simulink model "case7"  (R2024b)
settings: Solver=FixedStepAuto  StartTime=0  StopTime=1  FixedStep=1e-7  RelTol=1e-3
values from neighbouring files (symbols this model uses):
  SG_D_1_D = 0.01056    [IEEE9_case_parameters.m]    (also in case1_parameters.m; case2_parameters.m; case3_parameters.m; case4_parameters.m)
  SG_D_1_EnableSaturation = 0    [IEEE9_case_parameters.m]    (also in case1_parameters.m; case2_parameters.m; case3_parameters.m; case4_parameters.m)
  SG_D_1_f0 = 60    [IEEE9_case_parameters.m]    (also in case1_parameters.m; case2_parameters.m; case3_parameters.m; case4_parameters.m)
  SG_D_1_H = 7.5    [IEEE9_case_parameters.m]    (also in case1_parameters.m; case2_parameters.m; case3_parameters.m; case4_parameters.m)
  SG_D_1_K_A = 20    [IEEE9_case_parameters.m]    (also in case1_parameters.m; case2_parameters.m; case3_parameters.m; case4_parameters.m)
  SG_D_1_K_E = 1.000000e+1    (= 10)    [IEEE9_case_parameters.m]    (also in case1_parameters.m; case2_parameters.m; case3_parameters.m; case4_parameters.m)
  SG_D_1_K_F = 2.363    [IEEE9_case_parameters.m]    (also in case1_parameters.m; case2_parameters.m; case3_parameters.m; case4_parameters.m)
  SG_D_1_K_s = 0.5    [IEEE9_case_parameters.m]    (also in case1_parameters.m = 5; case2_parameters.m = 5; case3_parameters.m = 5; case4_parameters.m = 5)
  SG_D_1_R_a = 0.001088    [IEEE9_case_parameters.m]    (also in case1_parameters.m; case2_parameters.m; case3_parameters.m; case4_parameters.m)
  SG_D_1_S_A = 1    [IEEE9_case_parameters.m]    (also in case1_parameters.m; case2_parameters.m; case3_parameters.m; case4_parameters.m)
  SG_D_1_S_B = 0.103    [IEEE9_case_parameters.m]    (also in case1_parameters.m; case2_parameters.m; case3_parameters.m; case4_parameters.m)
  SG_D_1_S_N = 10.659857    [IEEE9_case_parameters.m]    (also in case1_parameters.m; case2_parameters.m; case3_parameters.m; case4_parameters.m)
  SG_D_1_SpeedPara = 200    [IEEE9_case_parameters.m]    (also in case1_parameters.m; case2_parameters.m; case3_parameters.m; case4_parameters.m)
  SG_D_1_T_0 = 0.720173    [IEEE9_case_parameters.m]    (also in case1_parameters.m = 0.755522; case2_parameters.m = 0.808931; case3_parameters.m = 0.869402; case4_parameters.m = 0.729316)
  SG_D_1_T_1 = 0.3    [IEEE9_case_parameters.m]    (also in case1_parameters.m; case2_parameters.m; case3_parameters.m; case4_parameters.m)
  SG_D_1_T_2 = 0.05    [IEEE9_case_parameters.m]    (also in case1_parameters.m; case2_parameters.m; case3_parameters.m; case4_parameters.m)
  SG_D_1_T_3 = 0.02    [IEEE9_case_parameters.m]    (also in case1_parameters.m; case2_parameters.m; case3_parameters.m; case4_parameters.m)
  SG_D_1_T_4 = 0.005    [IEEE9_case_parameters.m]    (also in case1_parameters.m; case2_parameters.m; case3_parameters.m; case4_parameters.m)
  SG_D_1_T_A = 0.02    [IEEE9_case_parameters.m]    (also in case1_parameters.m; case2_parameters.m; case3_parameters.m; case4_parameters.m)
  SG_D_1_T_dd = 8.000000e+0    (= 8)    [IEEE9_case_parameters.m]    (also in case1_parameters.m; case2_parameters.m; case3_parameters.m; case4_parameters.m)
  SG_D_1_T_ddd = 0.04    [IEEE9_case_parameters.m]    (also in case1_parameters.m; case2_parameters.m; case3_parameters.m; case4_parameters.m)
  SG_D_1_T_E = 0.314    [IEEE9_case_parameters.m]    (also in case1_parameters.m; case2_parameters.m; case3_parameters.m; case4_parameters.m)
  SG_D_1_T_F = 0.35    [IEEE9_case_parameters.m]    (also in case1_parameters.m; case2_parameters.m; case3_parameters.m; case4_parameters.m)
  SG_D_1_T_qd = 0.8    [IEEE9_case_parameters.m]    (also in case1_parameters.m; case2_parameters.m; case3_parameters.m; case4_parameters.m)
  SG_D_1_T_qdd = 0.02    [IEEE9_case_parameters.m]    (also in case1_parameters.m; case2_parameters.m; case3_parameters.m; case4_parameters.m)
  SG_D_1_T_speed = 0.1    [IEEE9_case_parameters.m]    (also in case1_parameters.m = 200; case2_parameters.m = 200; case3_parameters.m = 200; case4_parameters.m = 200)
  SG_D_1_T_w = 0.5    [IEEE9_case_parameters.m]    (also in case1_parameters.m; case2_parameters.m; case3_parameters.m; case4_parameters.m)
  SG_D_1_V_ref = 1.990276    [IEEE9_case_parameters.m]    (also in case1_parameters.m = 2.042296; case2_parameters.m = 2.051388; case3_parameters.m = 2.089584; case4_parameters.m = 2.01845)
  SG_D_1_w_ref = 376.991118    [IEEE9_case_parameters.m]    (also in case1_parameters.m; case2_parameters.m; case3_parameters.m; case4_parameters.m)
  SG_D_1_wb = 6.000000e+1    (= 60)    [IEEE9_case_parameters.m]    (also in case1_parameters.m; case2_parameters.m; case3_parameters.m; case4_parameters.m)
  SG_D_1_x_d = 1.9    [IEEE9_case_parameters.m]    (also in case1_parameters.m; case2_parameters.m; case3_parameters.m; case4_parameters.m)
  SG_D_1_x_dd = 0.302    [IEEE9_case_parameters.m]    (also in case1_parameters.m; case2_parameters.m; case3_parameters.m; case4_parameters.m)
  SG_D_1_x_ddd = 0.204    [IEEE9_case_parameters.m]    (also in case1_parameters.m; case2_parameters.m; case3_parameters.m; case4_parameters.m)
  SG_D_1_x_l = 0.05    [IEEE9_case_parameters.m]    (also in case1_parameters.m; case2_parameters.m; case3_parameters.m; case4_parameters.m)
  SG_D_1_x_q = 1.3    [IEEE9_case_parameters.m]    (also in case1_parameters.m; case2_parameters.m; case3_parameters.m; case4_parameters.m)
  SG_D_1_x_qd = 0.5    [IEEE9_case_parameters.m]    (also in case1_parameters.m; case2_parameters.m; case3_parameters.m; case4_parameters.m)
  SG_D_1_x_qdd = 0.3    [IEEE9_case_parameters.m]    (also in case1_parameters.m; case2_parameters.m; case3_parameters.m; case4_parameters.m)
  SG_D_2_D = 0.02    [IEEE9_case_parameters.m]    (also in case1_parameters.m; case2_parameters.m; case3_parameters.m; case4_parameters.m)
  SG_D_2_EnableSaturation = 0    [IEEE9_case_parameters.m]    (also in case1_parameters.m; case2_parameters.m; case3_parameters.m; case4_parameters.m)
  SG_D_2_f0 = 60    [IEEE9_case_parameters.m]    (also in case1_parameters.m; case2_parameters.m; case3_parameters.m; case4_parameters.m)
  SG_D_2_H = 8.000000e+0    (= 8)    [IEEE9_case_parameters.m]    (also in case1_parameters.m; case2_parameters.m; case3_parameters.m; case4_parameters.m)
  SG_D_2_K_A = 20    [IEEE9_case_parameters.m]    (also in case1_parameters.m; case2_parameters.m; case3_parameters.m; case4_parameters.m)
  SG_D_2_K_E = 1.000000e+1    (= 10)    [IEEE9_case_parameters.m]    (also in case1_parameters.m; case2_parameters.m; case3_parameters.m; case4_parameters.m)
  SG_D_2_K_F = 2.363    [IEEE9_case_parameters.m]    (also in case1_parameters.m; case2_parameters.m; case3_parameters.m; case4_parameters.m)
  SG_D_2_K_s = 0.5    [IEEE9_case_parameters.m]    (also in case1_parameters.m = 4; case2_parameters.m = 4; case3_parameters.m = 4; case4_parameters.m = 4)
  SG_D_2_R_a = 0.001088    [IEEE9_case_parameters.m]    (also in case1_parameters.m; case2_parameters.m; case3_parameters.m; case4_parameters.m)
  SG_D_2_S_A = 1    [IEEE9_case_parameters.m]    (also in case1_parameters.m; case2_parameters.m; case3_parameters.m; case4_parameters.m)
  SG_D_2_S_B = 0.103    [IEEE9_case_parameters.m]    (also in case1_parameters.m; case2_parameters.m; case3_parameters.m; case4_parameters.m)
  SG_D_2_S_N = 10.659857    [IEEE9_case_parameters.m]    (also in case1_parameters.m; case2_parameters.m; case3_parameters.m; case4_parameters.m)
  SG_D_2_SpeedPara = 200    [IEEE9_case_parameters.m]    (also in case1_parameters.m; case2_parameters.m; case3_parameters.m; case4_parameters.m)
  SG_D_2_T_0 = 1.632913    [IEEE9_case_parameters.m]    (also in case1_parameters.m = 1.632925; case2_parameters.m = 1.632915; case3_parameters.m = 1.632914; case4_parameters.m = 1.632927)
  SG_D_2_T_1 = 0.2    [IEEE9_case_parameters.m]    (also in case1_parameters.m; case2_parameters.m; case3_parameters.m; case4_parameters.m)
  SG_D_2_T_2 = 0.05    [IEEE9_case_parameters.m]    (also in case1_parameters.m; case2_parameters.m; case3_parameters.m; case4_parameters.m)
  SG_D_2_T_3 = 0.02    [IEEE9_case_parameters.m]    (also in case1_parameters.m; case2_parameters.m; case3_parameters.m; case4_parameters.m)
  SG_D_2_T_4 = 0.005    [IEEE9_case_parameters.m]    (also in case1_parameters.m; case2_parameters.m; case3_parameters.m; case4_parameters.m)
  SG_D_2_T_A = 0.02    [IEEE9_case_parameters.m]    (also in case1_parameters.m; case2_parameters.m; case3_parameters.m; case4_parameters.m)
  SG_D_2_T_dd = 7.9    [IEEE9_case_parameters.m]    (also in case1_parameters.m; case2_parameters.m; case3_parameters.m; case4_parameters.m)
  SG_D_2_T_ddd = 0.04    [IEEE9_case_parameters.m]    (also in case1_parameters.m; case2_parameters.m; case3_parameters.m; case4_parameters.m)
  SG_D_2_T_E = 0.314    [IEEE9_case_parameters.m]    (also in case1_parameters.m; case2_parameters.m; case3_parameters.m; case4_parameters.m)
  SG_D_2_T_F = 0.35    [IEEE9_case_parameters.m]    (also in case1_parameters.m; case2_parameters.m; case3_parameters.m; case4_parameters.m)
  SG_D_2_T_qd = 0.8    [IEEE9_case_parameters.m]    (also in case1_parameters.m; case2_parameters.m; case3_parameters.m; case4_parameters.m)
  SG_D_2_T_qdd = 0.015    [IEEE9_case_parameters.m]    (also in case1_parameters.m; case2_parameters.m; case3_parameters.m; case4_parameters.m)
  SG_D_2_T_speed = 0.1    [IEEE9_case_parameters.m]    (also in case1_parameters.m = 150; case2_parameters.m = 150; case3_parameters.m = 150; case4_parameters.m = 150)
  SG_D_2_T_w = 0.35    [IEEE9_case_parameters.m]    (also in case1_parameters.m; case2_parameters.m; case3_parameters.m; case4_parameters.m)
  SG_D_2_V_ref = 2.58547    [IEEE9_case_parameters.m]    (also in case1_parameters.m = 2.597896; case2_parameters.m = 2.587136; case3_parameters.m = 2.586042; case4_parameters.m = 2.599679)
  SG_D_2_w_ref = 376.991118    [IEEE9_case_parameters.m]    (also in case1_parameters.m; case2_parameters.m; case3_parameters.m; case4_parameters.m)
  SG_D_2_wb = 6.000000e+1    (= 60)    [IEEE9_case_parameters.m]    (also in case1_parameters.m; case2_parameters.m; case3_parameters.m; case4_parameters.m)
  SG_D_2_x_d = 1.8    [IEEE9_case_parameters.m]    (also in case1_parameters.m; case2_parameters.m; case3_parameters.m; case4_parameters.m)
  SG_D_2_x_dd = 0.302    [IEEE9_case_parameters.m]    (also in case1_parameters.m; case2_parameters.m; case3_parameters.m; case4_parameters.m)
  SG_D_2_x_ddd = 0.204    [IEEE9_case_parameters.m]    (also in case1_parameters.m; case2_parameters.m; case3_parameters.m; case4_parameters.m)
  SG_D_2_x_l = 0.05    [IEEE9_case_parameters.m]    (also in case1_parameters.m; case2_parameters.m; case3_parameters.m; case4_parameters.m)
  SG_D_2_x_q = 1.25    [IEEE9_case_parameters.m]    (also in case1_parameters.m; case2_parameters.m; case3_parameters.m; case4_parameters.m)
  SG_D_2_x_qd = 0.5    [IEEE9_case_parameters.m]    (also in case1_parameters.m; case2_parameters.m; case3_parameters.m; case4_parameters.m)
  SG_D_2_x_qdd = 0.3    [IEEE9_case_parameters.m]    (also in case1_parameters.m; case2_parameters.m; case3_parameters.m; case4_parameters.m)
  SG_D_3_D = 0.02    [IEEE9_case_parameters.m]    (also in case1_parameters.m; case2_parameters.m; case3_parameters.m; case4_parameters.m)
  SG_D_3_EnableSaturation = 0    [IEEE9_case_parameters.m]    (also in case1_parameters.m; case2_parameters.m; case3_parameters.m; case4_parameters.m)
  SG_D_3_f0 = 60    [IEEE9_case_parameters.m]    (also in case1_parameters.m; case2_parameters.m; case3_parameters.m; case4_parameters.m)
  SG_D_3_H = 7.7    [IEEE9_case_parameters.m]    (also in case1_parameters.m; case2_parameters.m; case3_parameters.m; case4_parameters.m)
  SG_D_3_K_A = 20    [IEEE9_case_parameters.m]    (also in case1_parameters.m; case2_parameters.m; case3_parameters.m; case4_parameters.m)
  SG_D_3_K_E = 1.000000e+1    (= 10)    [IEEE9_case_parameters.m]    (also in case1_parameters.m; case2_parameters.m; case3_parameters.m; case4_parameters.m)
  SG_D_3_K_F = 2.363    [IEEE9_case_parameters.m]    (also in case1_parameters.m; case2_parameters.m; case3_parameters.m; case4_parameters.m)
  SG_D_3_K_s = 0.2    [IEEE9_case_parameters.m]    (also in case1_parameters.m = 2; case2_parameters.m = 2; case3_parameters.m = 2; case4_parameters.m = 2)
  SG_D_3_R_a = 0.001088    [IEEE9_case_parameters.m]    (also in case1_parameters.m; case2_parameters.m; case3_parameters.m; case4_parameters.m)
  SG_D_3_S_A = 1    [IEEE9_case_parameters.m]    (also in case1_parameters.m; case2_parameters.m; case3_parameters.m; case4_parameters.m)
  SG_D_3_S_B = 0.103    [IEEE9_case_parameters.m]    (also in case1_parameters.m; case2_parameters.m; case3_parameters.m; case4_parameters.m)
  SG_D_3_S_N = 10.659857    [IEEE9_case_parameters.m]    (also in case1_parameters.m; case2_parameters.m; case3_parameters.m; case4_parameters.m)
  SG_D_3_SpeedPara = 200    [IEEE9_case_parameters.m]    (also in case1_parameters.m; case2_parameters.m; case3_parameters.m; case4_parameters.m)
  SG_D_3_T_0 = 0.850788    [IEEE9_case_parameters.m]    (also in case1_parameters.m = 0.850786; case2_parameters.m = 0.850787; case3_parameters.m; case4_parameters.m = 0.850786)
  SG_D_3_T_1 = 0.2    [IEEE9_case_parameters.m]    (also in case1_parameters.m; case2_parameters.m; case3_parameters.m; case4_parameters.m)
  SG_D_3_T_2 = 0.05    [IEEE9_case_parameters.m]    (also in case1_parameters.m; case2_parameters.m; case3_parameters.m; case4_parameters.m)
  SG_D_3_T_3 = 0.02    [IEEE9_case_parameters.m]    (also in case1_parameters.m; case2_parameters.m; case3_parameters.m; case4_parameters.m)
  SG_D_3_T_4 = 0.005    [IEEE9_case_parameters.m]    (also in case1_parameters.m; case2_parameters.m; case3_parameters.m; case4_parameters.m)
  SG_D_3_T_A = 0.02    [IEEE9_case_parameters.m]    (also in case1_parameters.m; case2_parameters.m; case3_parameters.m; case4_parameters.m)
  SG_D_3_T_dd = 8.1    [IEEE9_case_parameters.m]    (also in case1_parameters.m; case2_parameters.m; case3_parameters.m; case4_parameters.m)
  SG_D_3_T_ddd = 0.04    [IEEE9_case_parameters.m]    (also in case1_parameters.m; case2_parameters.m; case3_parameters.m; case4_parameters.m)
  SG_D_3_T_E = 0.314    [IEEE9_case_parameters.m]    (also in case1_parameters.m; case2_parameters.m; case3_parameters.m; case4_parameters.m)
  SG_D_3_T_F = 0.35    [IEEE9_case_parameters.m]    (also in case1_parameters.m; case2_parameters.m; case3_parameters.m; case4_parameters.m)
  SG_D_3_T_qd = 0.8    [IEEE9_case_parameters.m]    (also in case1_parameters.m; case2_parameters.m; case3_parameters.m; case4_parameters.m)
  SG_D_3_T_qdd = 0.015    [IEEE9_case_parameters.m]    (also in case1_parameters.m; case2_parameters.m; case3_parameters.m; case4_parameters.m)
  SG_D_3_T_speed = 0.1    [IEEE9_case_parameters.m]    (also in case1_parameters.m = 180; case2_parameters.m = 180; case3_parameters.m = 180; case4_parameters.m = 180)
  SG_D_3_T_w = 0.4    [IEEE9_case_parameters.m]    (also in case1_parameters.m; case2_parameters.m; case3_parameters.m; case4_parameters.m)
  SG_D_3_V_ref = 1.892727    [IEEE9_case_parameters.m]    (also in case1_parameters.m = 1.906439; case2_parameters.m = 1.895535; case3_parameters.m = 1.892105; case4_parameters.m = 1.906598)
  SG_D_3_w_ref = 376.991118    [IEEE9_case_parameters.m]    (also in case1_parameters.m; case2_parameters.m; case3_parameters.m; case4_parameters.m)
  SG_D_3_wb = 6.000000e+1    (= 60)    [IEEE9_case_parameters.m]    (also in case1_parameters.m; case2_parameters.m; case3_parameters.m; case4_parameters.m)
  SG_D_3_x_d = 1.85    [IEEE9_case_parameters.m]    (also in case1_parameters.m; case2_parameters.m; case3_parameters.m; case4_parameters.m)
  SG_D_3_x_dd = 0.302    [IEEE9_case_parameters.m]    (also in case1_parameters.m; case2_parameters.m; case3_parameters.m; case4_parameters.m)
  SG_D_3_x_ddd = 0.204    [IEEE9_case_parameters.m]    (also in case1_parameters.m; case2_parameters.m; case3_parameters.m; case4_parameters.m)
  SG_D_3_x_l = 0.05    [IEEE9_case_parameters.m]    (also in case1_parameters.m; case2_parameters.m; case3_parameters.m; case4_parameters.m)
  SG_D_3_x_q = 1.2    [IEEE9_case_parameters.m]    (also in case1_parameters.m; case2_parameters.m; case3_parameters.m; case4_parameters.m)
  SG_D_3_x_qd = 0.5    [IEEE9_case_parameters.m]    (also in case1_parameters.m; case2_parameters.m; case3_parameters.m; case4_parameters.m)
  SG_D_3_x_qdd = 0.3    [IEEE9_case_parameters.m]    (also in case1_parameters.m; case2_parameters.m; case3_parameters.m; case4_parameters.m)
(part 1 of 12)
settings Model: Creator=Greg  LastModifiedBy=Greg

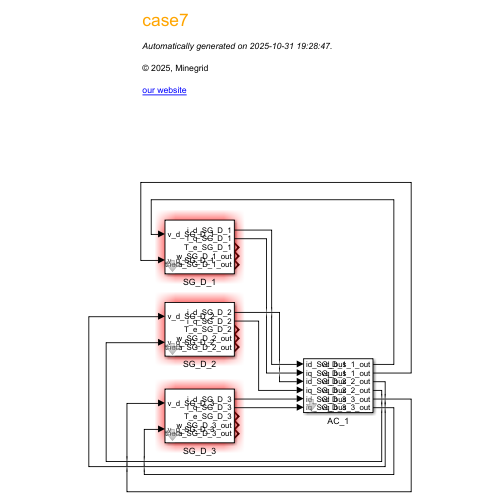
[thumbnail: Simulink's stored preview of the top-level diagram]
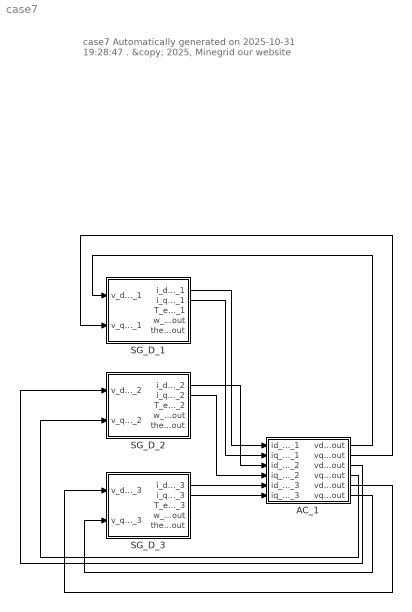
== system case7 ==
  note: case7
      | Automatically generated on 2025-10-31 19:28:47 .
      | &copy; 2025, Minegrid
      | our website
  AC_1 : Subsystem  mask(AC_1){}
      mask help: Parameters Interface of AC_1
  SG_D_1 : Subsystem  mask(SG_D_1){T_0=SG_D_1_T_0, w_ref=SG_D_1_w_ref, V_ref=SG_D_1_V_ref, x_d=SG_D_1_x_d, x_dd=SG_D_1_x_dd, x_ddd=SG_D_1_x_ddd, x_q=SG_D_1_x_q, x_qd=SG_D_1_x_qd, x_qdd=SG_D_1_x_qdd, x_l=SG_D_1_x_l, R_a=SG_D_1_R_a, T_dd=SG_D_1_T_dd, T_ddd=SG_D_1_T_ddd, T_qd=SG_D_1_T_qd, T_qdd=SG_D_1_T_qdd, H=SG_D_1_H, D=SG_D_1_D, SpeedPara=SG_D_1_SpeedPara, K_A=SG_D_1_K_A, EnableSaturation=SG_D_1_EnableSaturation, f0=SG_D_1_f0, T_speed=SG_D_1_T_speed, T_E=SG_D_1_T_E, T_A=SG_D_1_T_A, T_F=SG_D_1_T_F, K_E=SG_D_1_K_E, K_F=SG_D_1_K_F, K_s=SG_D_1_K_s, T_1=SG_D_1_T_1, T_2=SG_D_1_T_2, T_3=SG_D_1_T_3, T_4=SG_D_1_T_4, T_w=SG_D_1_T_w, wb=SG_D_1_wb, S_A=SG_D_1_S_A, S_B=SG_D_1_S_B, S_N=SG_D_1_S_N}
      mask help: Parameters Interface of SG_D_1
  SG_D_2 : Subsystem  mask(SG_D_2){T_0=SG_D_2_T_0, w_ref=SG_D_2_w_ref, V_ref=SG_D_2_V_ref, x_d=SG_D_2_x_d, x_dd=SG_D_2_x_dd, x_ddd=SG_D_2_x_ddd, x_q=SG_D_2_x_q, x_qd=SG_D_2_x_qd, x_qdd=SG_D_2_x_qdd, x_l=SG_D_2_x_l, R_a=SG_D_2_R_a, T_dd=SG_D_2_T_dd, T_ddd=SG_D_2_T_ddd, T_qd=SG_D_2_T_qd, T_qdd=SG_D_2_T_qdd, H=SG_D_2_H, D=SG_D_2_D, SpeedPara=SG_D_2_SpeedPara, K_A=SG_D_2_K_A, EnableSaturation=SG_D_2_EnableSaturation, f0=SG_D_2_f0, T_speed=SG_D_2_T_speed, T_E=SG_D_2_T_E, T_A=SG_D_2_T_A, T_F=SG_D_2_T_F, K_E=SG_D_2_K_E, K_F=SG_D_2_K_F, K_s=SG_D_2_K_s, T_1=SG_D_2_T_1, T_2=SG_D_2_T_2, T_3=SG_D_2_T_3, T_4=SG_D_2_T_4, T_w=SG_D_2_T_w, wb=SG_D_2_wb, S_A=SG_D_2_S_A, S_B=SG_D_2_S_B, S_N=SG_D_2_S_N}
      mask help: Parameters Interface of SG_D_2
  SG_D_3 : Subsystem  mask(SG_D_3){T_0=SG_D_3_T_0, w_ref=SG_D_3_w_ref, V_ref=SG_D_3_V_ref, x_d=SG_D_3_x_d, x_dd=SG_D_3_x_dd, x_ddd=SG_D_3_x_ddd, x_q=SG_D_3_x_q, x_qd=SG_D_3_x_qd, x_qdd=SG_D_3_x_qdd, x_l=SG_D_3_x_l, R_a=SG_D_3_R_a, T_dd=SG_D_3_T_dd, T_ddd=SG_D_3_T_ddd, T_qd=SG_D_3_T_qd, T_qdd=SG_D_3_T_qdd, H=SG_D_3_H, D=SG_D_3_D, SpeedPara=SG_D_3_SpeedPara, K_A=SG_D_3_K_A, EnableSaturation=SG_D_3_EnableSaturation, f0=SG_D_3_f0, T_speed=SG_D_3_T_speed, T_E=SG_D_3_T_E, T_A=SG_D_3_T_A, T_F=SG_D_3_T_F, K_E=SG_D_3_K_E, K_F=SG_D_3_K_F, K_s=SG_D_3_K_s, T_1=SG_D_3_T_1, T_2=SG_D_3_T_2, T_3=SG_D_3_T_3, T_4=SG_D_3_T_4, T_w=SG_D_3_T_w, wb=SG_D_3_wb, S_A=SG_D_3_S_A, S_B=SG_D_3_S_B, S_N=SG_D_3_S_N}
      mask help: Parameters Interface of SG_D_3
  wires:
  SG_D_2/2(i_q_SG_D_2) -> AC_1/4(iq_SG_D_2)
  SG_D_1/2(i_q_SG_D_1) -> AC_1/2(iq_SG_D_1)
  SG_D_1/1(i_d_SG_D_1) -> AC_1/1(id_SG_D_1)
  SG_D_2/1(i_d_SG_D_2) -> AC_1/3(id_SG_D_2)
  AC_1/1(vd_bus_1_out) -> SG_D_1/1(v_d_SG_D_1)
  SG_D_3/1(i_d_SG_D_3) -> AC_1/5(id_SG_D_3)
  AC_1/2(vq_bus_1_out) -> SG_D_1/2(v_q_SG_D_1)
  SG_D_3/2(i_q_SG_D_3) -> AC_1/6(iq_SG_D_3)
  AC_1/3(vd_bus_2_out) -> SG_D_2/1(v_d_SG_D_2)
  AC_1/4(vq_bus_2_out) -> SG_D_2/2(v_q_SG_D_2)
  AC_1/5(vd_bus_3_out) -> SG_D_3/1(v_d_SG_D_3)
  AC_1/6(vq_bus_3_out) -> SG_D_3/2(v_q_SG_D_3)

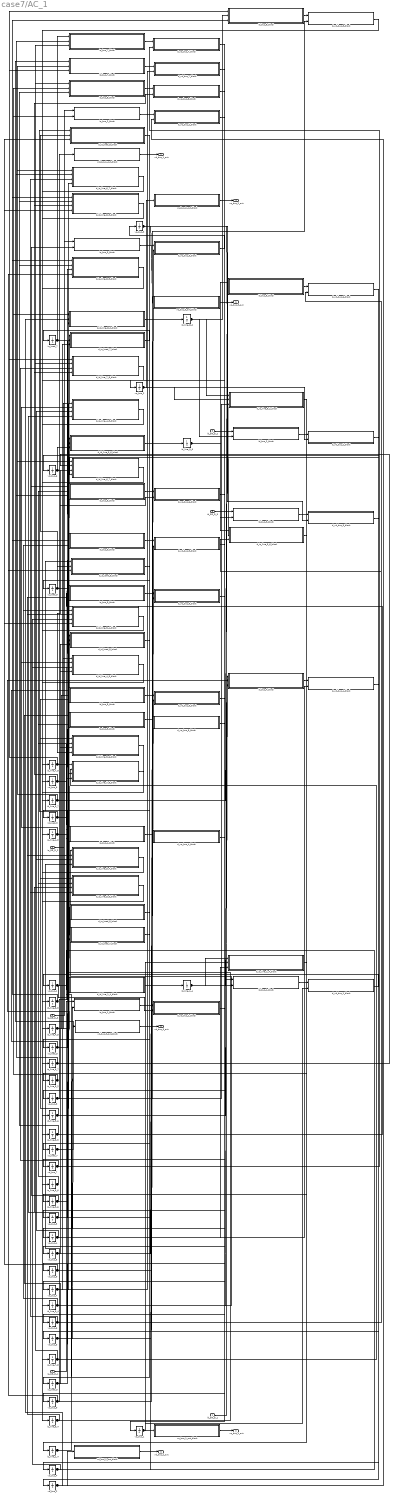
== system case7/AC_1 ==
  id_SG_D_1 : Inport
  iq_SG_D_1 : Inport  Port=2
  id_SG_D_2 : Inport  Port=3
  iq_SG_D_2 : Inport  Port=4
  id_SG_D_3 : Inport  Port=5
  iq_SG_D_3 : Inport  Port=6
  d_id_line_1_4_block : Subsystem
  d_id_line_3_6_block : Subsystem
  d_id_line_4_5_block : Subsystem
  d_id_line_5_6_block : Subsystem
  d_id_line_6_7_block : Subsystem
  d_id_line_7_8_block : Subsystem
  d_id_line_8_2_block : Subsystem
  d_id_line_8_9_block : Subsystem
  d_id_line_9_4_block : Subsystem
  d_id_load_5_block : Subsystem
  d_id_load_7_block : Subsystem
  d_id_load_9_block : Subsystem
  d_iq_line_1_4_block : Subsystem
  d_iq_line_3_6_block : Subsystem
  d_iq_line_4_5_block : Subsystem
  d_iq_line_5_6_block : Subsystem
  d_iq_line_6_7_block : Subsystem
  d_iq_line_7_8_block : Subsystem
  d_iq_line_8_2_block : Subsystem
  d_iq_line_8_9_block : Subsystem
  d_iq_line_9_4_block : Subsystem
  d_iq_load_5_block : Subsystem
  d_iq_load_7_block : Subsystem
  d_iq_load_9_block : Subsystem
  d_vd_bus_1_block : Subsystem
  d_vd_bus_2_block : Subsystem
  d_vd_bus_3_block : Subsystem
  d_vd_bus_4_block : Subsystem
  d_vd_bus_5_block : Subsystem
  d_vd_bus_6_block : Subsystem
  d_vd_bus_7_block : Subsystem
  d_vd_bus_8_block : Subsystem
  d_vd_bus_9_block : Subsystem
  d_vq_bus_1_block : Subsystem
  d_vq_bus_2_block : Subsystem
  d_vq_bus_3_block : Subsystem
  d_vq_bus_4_block : Subsystem
  d_vq_bus_5_block : Subsystem
  d_vq_bus_6_block : Subsystem
  d_vq_bus_7_block : Subsystem
  d_vq_bus_8_block : Subsystem
  d_vq_bus_9_block : Subsystem
  id_bus_1_block : Subsystem
  id_bus_2_block : Subsystem
  id_bus_3_block : Subsystem
  id_bus_4_block : Subsystem
  id_bus_5_block : Subsystem
  id_bus_6_block : Subsystem
  id_bus_7_block : Subsystem
  id_bus_8_block : Subsystem
  id_bus_9_block : Subsystem
  id_line_1_4 : Integrator  InitialCondition=0.7046
  id_line_3_6 : Integrator  InitialCondition=0.841
  id_line_4_5 : Integrator  InitialCondition=0.3014
  id_line_5_6 : Integrator  InitialCondition=-0.609
  id_line_6_7 : Integrator  InitialCondition=0.2421
  id_line_7_8 : Integrator  InitialCondition=-0.766
  id_line_8_2 : Integrator  InitialCondition=-1.6245
  id_line_8_9 : Integrator  InitialCondition=0.874
  id_line_9_4 : Integrator  InitialCondition=-0.3964
  id_load_5 : Integrator  InitialCondition=0.8929736913465931
  id_load_7 : Integrator  InitialCondition=1.0103745512612274
  id_load_9 : Integrator  InitialCondition=1.2530677383718292
  iq_bus_1_block : Subsystem
  iq_bus_2_block : Subsystem
  iq_bus_3_block : Subsystem
  iq_bus_4_block : Subsystem
  iq_bus_5_block : Subsystem
  iq_bus_6_block : Subsystem
  iq_bus_7_block : Subsystem
  iq_bus_8_block : Subsystem
  iq_bus_9_block : Subsystem
  iq_line_1_4 : Integrator  InitialCondition=-0.1877
  iq_line_3_6 : Integrator  InitialCondition=0.1412
  iq_line_4_5 : Integrator  InitialCondition=-0.0675
  iq_line_5_6 : Integrator  InitialCondition=0.0199
  iq_line_6_7 : Integrator  InitialCondition=-0.1237
  iq_line_7_8 : Integrator  InitialCondition=0.0069
  iq_line_8_2 : Integrator  InitialCondition=-0.1716
  iq_line_8_9 : Integrator  InitialCondition=-0.0481
  iq_line_9_4 : Integrator  InitialCondition=0.2855
  iq_load_5 : Integrator  InitialCondition=-0.3396268514243827
  iq_load_7 : Integrator  InitialCondition=-0.30769449147731925
  iq_load_9 : Integrator  InitialCondition=-0.5651600829422596
  vd_bus_1 : Integrator  InitialCondition=1.0
  vd_bus_1_out_block : Subsystem
  vd_bus_2 : Integrator  InitialCondition=0.9854656089996572
  vd_bus_2_out_block : Subsystem
  vd_bus_3 : Integrator  InitialCondition=0.9963648946924322
  vd_bus_3_out_block : Subsystem
  vd_bus_4 : Integrator  InitialCondition=0.9891468763636446
  vd_bus_5 : Integrator  InitialCondition=0.977867619882352
  vd_bus_6 : Integrator  InitialCondition=1.0046719033619074
  vd_bus_7 : Integrator  InitialCondition=0.9893152199851127
  vd_bus_8 : Integrator  InitialCondition=0.996231319283822
  vd_bus_9 : Integrator  InitialCondition=0.9608859398821573
  vq_bus_1 : Integrator  InitialCondition=0.0
  vq_bus_1_out_block : Subsystem
  vq_bus_2 : Integrator  InitialCondition=0.16987505255020435
  vq_bus_2_out_block : Subsystem
  vq_bus_3 : Integrator  InitialCondition=0.08518800751595623
  vq_bus_3_out_block : Subsystem
  vq_bus_4 : Integrator  InitialCondition=-0.040732947337366425
  vq_bus_5 : Integrator  InitialCondition=-0.06742985670686191
  vq_bus_6 : Integrator  InitialCondition=0.035721536791196516
  vq_bus_7 : Integrator  InitialCondition=0.012674842274998602
  vq_bus_8 : Integrator  InitialCondition=0.06797079213073709
  vq_bus_9 : Integrator  InitialCondition=-0.07173809262590466
  vd_bus_1_out : Outport
  vq_bus_1_out : Outport  Port=2
  vd_bus_2_out : Outport  Port=3
  vq_bus_2_out : Outport  Port=4
  vd_bus_3_out : Outport  Port=5
  vq_bus_3_out : Outport  Port=6
  wires:
  vd_bus_9/1 -> d_id_load_9_block/3(State_vd_bus_9_88276), d_id_line_9_4_block/4(State_vd_bus_9_20c24), d_vq_bus_9_block/2(State_vd_bus_9_2f8b2), d_id_line_8_9_block/4(State_vd_bus_9_2283c)
  d_id_line_5_6_block/1(Blockout_d_id_line_5_6_fc4e7) -> id_line_5_6/1
  d_iq_load_5_block/1(Blockout_d_iq_load_5_d6271) -> iq_load_5/1
  id_line_4_5/1 -> id_bus_4_block/2(State_id_line_4_5_64512), d_id_line_4_5_block/1(State_id_line_4_5_e6f56), id_bus_5_block/2(State_id_line_4_5_aeb7d), d_iq_line_4_5_block/1(State_id_line_4_5_fca51)
  id_bus_6_block/1(Blockout_id_bus_6_34f1f) -> d_vd_bus_6_block/1(Alge_id_bus_6_09be4)
  d_id_load_7_block/1(Blockout_d_id_load_7_72daa) -> id_load_7/1
  iq_bus_6_block/1(Blockout_iq_bus_6_0cb61) -> d_vq_bus_6_block/1(Alge_iq_bus_6_c1a18)
  d_vq_bus_2_block/1(Blockout_d_vq_bus_2_220e4) -> vq_bus_2/1
  d_id_line_1_4_block/1(Blockout_d_id_line_1_4_c51d9) -> id_line_1_4/1
  vq_bus_2_out_block/1(Blockout_vq_bus_2_out_5c378) -> vq_bus_2_out/1
  iq_SG_D_3/1 -> iq_bus_3_block/1(Input_iq_SG_D_3_c42e5)
  d_vq_bus_4_block/1(Blockout_d_vq_bus_4_54be8) -> vq_bus_4/1
  iq_bus_9_block/1(Blockout_iq_bus_9_80b8d) -> d_vq_bus_9_block/1(Alge_iq_bus_9_a8f96)
  vd_bus_3_out_block/1(Blockout_vd_bus_3_out_587ae) -> vd_bus_3_out/1
  d_iq_line_8_2_block/1(Blockout_d_iq_line_8_2_76ae2) -> iq_line_8_2/1
  d_vd_bus_4_block/1(Blockout_d_vd_bus_4_77c2e) -> vd_bus_4/1
  id_SG_D_3/1 -> id_bus_3_block/1(Input_id_SG_D_3_5761d)
  d_vq_bus_7_block/1(Blockout_d_vq_bus_7_c9af2) -> vq_bus_7/1
  iq_bus_3_block/1(Blockout_iq_bus_3_7920f) -> d_vq_bus_3_block/1(Alge_iq_bus_3_bf354)
  id_load_5/1 -> d_iq_load_5_block/1(State_id_load_5_99883), id_bus_5_block/1(State_id_load_5_a1fc8), d_id_load_5_block/1(State_id_load_5_77b25)
  iq_line_8_2/1 -> d_id_line_8_2_block/1(State_iq_line_8_2_8eb85), iq_bus_2_block/2(State_iq_line_8_2_f6d21), iq_bus_8_block/2(State_iq_line_8_2_4ece4)
  iq_bus_1_block/1(Blockout_iq_bus_1_23a9f) -> d_vq_bus_1_block/1(Alge_iq_bus_1_697df)
  iq_SG_D_2/1 -> iq_bus_2_block/1(Input_iq_SG_D_2_9dccc)
  d_id_line_4_5_block/1(Blockout_d_id_line_4_5_dc71b) -> id_line_4_5/1
  id_SG_D_2/1 -> id_bus_2_block/1(Input_id_SG_D_2_cbeb2)
  id_bus_9_block/1(Blockout_id_bus_9_4ad6a) -> d_vd_bus_9_block/1(Alge_id_bus_9_c43c1)
  iq_SG_D_1/1 -> iq_bus_1_block/1(Input_iq_SG_D_1_419da)
  id_bus_1_block/1(Blockout_id_bus_1_e0036) -> d_vd_bus_1_block/1(Alge_id_bus_1_aedfe)
  id_line_1_4/1 -> id_bus_1_block/2(State_id_line_1_4_aab97), id_bus_4_block/1(State_id_line_1_4_3a3fb), d_iq_line_1_4_block/1(State_id_line_1_4_2037f)
  id_SG_D_1/1 -> id_bus_1_block/1(Input_id_SG_D_1_eabc6)
  id_line_8_9/1 -> id_bus_8_block/3(State_id_line_8_9_6c8e7), d_id_line_8_9_block/1(State_id_line_8_9_6c653), id_bus_9_block/2(State_id_line_8_9_50722), d_iq_line_8_9_block/1(State_id_line_8_9_ece40)
  d_id_line_3_6_block/1(Blockout_d_id_line_3_6_3d598) -> id_line_3_6/1
  d_id_line_8_2_block/1(Blockout_d_id_line_8_2_4b586) -> id_line_8_2/1
  vq_bus_3_out_block/1(Blockout_vq_bus_3_out_91852) -> vq_bus_3_out/1
  iq_bus_8_block/1(Blockout_iq_bus_8_3d53c) -> d_vq_bus_8_block/1(Alge_iq_bus_8_b3710)
  id_line_7_8/1 -> id_bus_8_block/1(State_id_line_7_8_e0e98), id_bus_7_block/3(State_id_line_7_8_244b4), d_id_line_7_8_block/1(State_id_line_7_8_0f689), d_iq_line_7_8_block/1(State_id_line_7_8_167a8)
  id_bus_3_block/1(Blockout_id_bus_3_ffcf5) -> d_vd_bus_3_block/1(Alge_id_bus_3_35d15)
  id_bus_8_block/1(Blockout_id_bus_8_dcf1d) -> d_vd_bus_8_block/1(Alge_id_bus_8_725a0)
  iq_bus_7_block/1(Blockout_iq_bus_7_f78e5) -> d_vq_bus_7_block/1(Alge_iq_bus_7_6c77e)
  iq_load_7/1 -> d_id_load_7_block/2(State_iq_load_7_dd7e6), d_iq_load_7_block/2(State_iq_load_7_999fa), iq_bus_7_block/1(State_iq_load_7_cacac)
  id_bus_7_block/1(Blockout_id_bus_7_f40f2) -> d_vd_bus_7_block/1(Alge_id_bus_7_a194e)
  iq_line_6_7/1 -> d_iq_line_6_7_block/2(State_iq_line_6_7_8e035), iq_bus_6_block/3(State_iq_line_6_7_e327a), d_id_line_6_7_block/2(State_iq_line_6_7_c6725), iq_bus_7_block/2(State_iq_line_6_7_1e244)
  iq_line_8_9/1 -> d_id_line_8_9_block/2(State_iq_line_8_9_a7084), iq_bus_8_block/3(State_iq_line_8_9_62274), iq_bus_9_block/2(State_iq_line_8_9_e9f4e), d_iq_line_8_9_block/2(State_iq_line_8_9_7b378)
  iq_bus_5_block/1(Blockout_iq_bus_5_1d005) -> d_vq_bus_5_block/1(Alge_iq_bus_5_edb30)
  id_bus_5_block/1(Blockout_id_bus_5_d8728) -> d_vd_bus_5_block/1(Alge_id_bus_5_39b8d)
  id_line_6_7/1 -> d_id_line_6_7_block/1(State_id_line_6_7_8b489), d_iq_line_6_7_block/1(State_id_line_6_7_f0a87), id_bus_6_block/3(State_id_line_6_7_41759), id_bus_7_block/2(State_id_line_6_7_22f92)
  id_bus_2_block/1(Blockout_id_bus_2_1dfd8) -> d_vd_bus_2_block/1(Alge_id_bus_2_e0197)
  iq_bus_4_block/1(Blockout_iq_bus_4_5b7f0) -> d_vq_bus_4_block/1(Alge_iq_bus_4_08719)
  id_load_7/1 -> d_iq_load_7_block/1(State_id_load_7_23b97), id_bus_7_block/1(State_id_load_7_264fa), d_id_load_7_block/1(State_id_load_7_f12d4)
  id_bus_4_block/1(Blockout_id_bus_4_096f4) -> d_vd_bus_4_block/1(Alge_id_bus_4_bf9d1)
  vd_bus_1_out_block/1(Blockout_vd_bus_1_out_c0c69) -> vd_bus_1_out/1
  vq_bus_1_out_block/1(Blockout_vq_bus_1_out_89e60) -> vq_bus_1_out/1
  iq_line_4_5/1 -> d_iq_line_4_5_block/2(State_iq_line_4_5_74164), iq_bus_4_block/2(State_iq_line_4_5_67a6b), iq_bus_5_block/2(State_iq_line_4_5_93363), d_id_line_4_5_block/2(State_iq_line_4_5_ed095)
  iq_load_5/1 -> d_id_load_5_block/2(State_iq_load_5_98165), iq_bus_5_block/1(State_iq_load_5_f86bc), d_iq_load_5_block/2(State_iq_load_5_ceced)
  id_line_9_4/1 -> id_bus_4_block/3(State_id_line_9_4_0d956), d_id_line_9_4_block/1(State_id_line_9_4_e74bb), id_bus_9_block/3(State_id_line_9_4_40117), d_iq_line_9_4_block/1(State_id_line_9_4_16341)
  iq_bus_2_block/1(Blockout_iq_bus_2_f07a2) -> d_vq_bus_2_block/1(Alge_iq_bus_2_6bd95)
  vd_bus_7/1 -> d_id_load_7_block/3(State_vd_bus_7_f2578), d_id_line_7_8_block/3(State_vd_bus_7_53355), d_id_line_6_7_block/4(State_vd_bus_7_b412f), d_vq_bus_7_block/2(State_vd_bus_7_c0edf)
  d_iq_line_7_8_block/1(Blockout_d_iq_line_7_8_6dc4f) -> iq_line_7_8/1
  vd_bus_2_out_block/1(Blockout_vd_bus_2_out_3aeaa) -> vd_bus_2_out/1
  iq_line_9_4/1 -> d_id_line_9_4_block/2(State_iq_line_9_4_d6adc), d_iq_line_9_4_block/2(State_iq_line_9_4_9816b), iq_bus_4_block/3(State_iq_line_9_4_bc136), iq_bus_9_block/3(State_iq_line_9_4_2d700)
  vq_bus_6/1 -> d_vd_bus_6_block/2(State_vq_bus_6_b4a62), d_iq_line_3_6_block/3(State_vq_bus_6_fdbe6), d_iq_line_5_6_block/4(State_vq_bus_6_cbe8b), d_iq_line_6_7_block/3(State_vq_bus_6_ef30c)
  d_iq_line_3_6_block/1(Blockout_d_iq_line_3_6_d1d92) -> iq_line_3_6/1
  d_id_line_8_9_block/1(Blockout_d_id_line_8_9_f11ed) -> id_line_8_9/1
  id_line_8_2/1 -> d_iq_line_8_2_block/1(State_id_line_8_2_6be89), id_bus_8_block/2(State_id_line_8_2_e2197), id_bus_2_block/2(State_id_line_8_2_ddc5d)
  d_id_line_9_4_block/1(Blockout_d_id_line_9_4_76f50) -> id_line_9_4/1
  vq_bus_5/1 -> d_vd_bus_5_block/2(State_vq_bus_5_e58cb), d_iq_load_5_block/3(State_vq_bus_5_33ca4), d_iq_line_4_5_block/4(State_vq_bus_5_c17cf), d_iq_line_5_6_block/3(State_vq_bus_5_06daf)
  d_id_line_6_7_block/1(Blockout_d_id_line_6_7_76637) -> id_line_6_7/1
  d_vq_bus_3_block/1(Blockout_d_vq_bus_3_782d4) -> vq_bus_3/1
  vd_bus_2/1 -> d_id_line_8_2_block/2(State_vd_bus_2_e858e), vd_bus_2_out_block/1(State_vd_bus_2_3d298), d_vq_bus_2_block/2(State_vd_bus_2_d11cb)
  vd_bus_4/1 -> d_vq_bus_4_block/2(State_vd_bus_4_858e6), d_id_line_1_4_block/3(State_vd_bus_4_026ae), d_id_line_4_5_block/3(State_vd_bus_4_76923), d_id_line_9_4_block/3(State_vd_bus_4_536cf)
  iq_line_7_8/1 -> d_id_line_7_8_block/2(State_iq_line_7_8_c6b57), d_iq_line_7_8_block/2(State_iq_line_7_8_7ac3b), iq_bus_7_block/3(State_iq_line_7_8_8c678), iq_bus_8_block/1(State_iq_line_7_8_8361f)
  vq_bus_3/1 -> vq_bus_3_out_block/1(State_vq_bus_3_a3a16), d_vd_bus_3_block/2(State_vq_bus_3_28960), d_iq_line_3_6_block/2(State_vq_bus_3_71d2c)
  vd_bus_8/1 -> d_vq_bus_8_block/2(State_vd_bus_8_12b43), d_id_line_8_2_block/3(State_vd_bus_8_0adbc), d_id_line_8_9_block/3(State_vd_bus_8_dd79d), d_id_line_7_8_block/4(State_vd_bus_8_337bf)
  id_line_3_6/1 -> d_iq_line_3_6_block/1(State_id_line_3_6_67359), id_bus_3_block/2(State_id_line_3_6_23ff0), id_bus_6_block/1(State_id_line_3_6_b6780)
  iq_line_3_6/1 -> d_id_line_3_6_block/1(State_iq_line_3_6_444c3), iq_bus_3_block/2(State_iq_line_3_6_82adc), iq_bus_6_block/1(State_iq_line_3_6_53eaa)
  iq_line_5_6/1 -> d_id_line_5_6_block/2(State_iq_line_5_6_26212), d_iq_line_5_6_block/2(State_iq_line_5_6_83796), iq_bus_5_block/3(State_iq_line_5_6_43169), iq_bus_6_block/2(State_iq_line_5_6_87c1e)
  id_line_5_6/1 -> d_id_line_5_6_block/1(State_id_line_5_6_f2138), d_iq_line_5_6_block/1(State_id_line_5_6_a603b), id_bus_5_block/3(State_id_line_5_6_7e5e7), id_bus_6_block/2(State_id_line_5_6_2d0d9)
  vd_bus_3/1 -> d_vq_bus_3_block/2(State_vd_bus_3_03f14), vd_bus_3_out_block/1(State_vd_bus_3_0fcd0), d_id_line_3_6_block/2(State_vd_bus_3_678dc)
  iq_line_1_4/1 -> d_id_line_1_4_block/1(State_iq_line_1_4_9d35a), iq_bus_4_block/1(State_iq_line_1_4_6e840), iq_bus_1_block/2(State_iq_line_1_4_cde6a)
  iq_load_9/1 -> d_iq_load_9_block/2(State_iq_load_9_40cec), iq_bus_9_block/1(State_iq_load_9_c0b16), d_id_load_9_block/2(State_iq_load_9_6adcd)
  id_load_9/1 -> d_id_load_9_block/1(State_id_load_9_96eb2), d_iq_load_9_block/1(State_id_load_9_f3e09), id_bus_9_block/1(State_id_load_9_bf11f)
  vd_bus_6/1 -> d_id_line_5_6_block/4(State_vd_bus_6_92612), d_id_line_3_6_block/3(State_vd_bus_6_3dc31), d_id_line_6_7_block/3(State_vd_bus_6_b4206), d_vq_bus_6_block/2(State_vd_bus_6_cf8cd)
  vq_bus_4/1 -> d_iq_line_1_4_block/3(State_vq_bus_4_e9fbb), d_vd_bus_4_block/2(State_vq_bus_4_a32d2), d_iq_line_9_4_block/3(State_vq_bus_4_2d516), d_iq_line_4_5_block/3(State_vq_bus_4_9a579)
  vq_bus_9/1 -> d_vd_bus_9_block/2(State_vq_bus_9_51ac1), d_iq_load_9_block/3(State_vq_bus_9_28711), d_iq_line_8_9_block/4(State_vq_bus_9_6e5a2), d_iq_line_9_4_block/4(State_vq_bus_9_6157d)
  vq_bus_1/1 -> d_vd_bus_1_block/2(State_vq_bus_1_b64b1), vq_bus_1_out_block/1(State_vq_bus_1_e6f2a), d_iq_line_1_4_block/2(State_vq_bus_1_e30e3)
  vq_bus_8/1 -> d_vd_bus_8_block/2(State_vq_bus_8_d9b83), d_iq_line_8_2_block/3(State_vq_bus_8_9749c), d_iq_line_7_8_block/4(State_vq_bus_8_c730a), d_iq_line_8_9_block/3(State_vq_bus_8_e5c45)
  vq_bus_7/1 -> d_vd_bus_7_block/2(State_vq_bus_7_51f84), d_iq_load_7_block/3(State_vq_bus_7_34020), d_iq_line_6_7_block/4(State_vq_bus_7_83713), d_iq_line_7_8_block/3(State_vq_bus_7_a194e)
  vd_bus_1/1 -> d_vq_bus_1_block/2(State_vd_bus_1_3d80d), vd_bus_1_out_block/1(State_vd_bus_1_3d051), d_id_line_1_4_block/2(State_vd_bus_1_07647)
  vd_bus_5/1 -> d_vq_bus_5_block/2(State_vd_bus_5_1db70), d_id_load_5_block/3(State_vd_bus_5_6eea2), d_id_line_4_5_block/4(State_vd_bus_5_748a8), d_id_line_5_6_block/3(State_vd_bus_5_5d5fa)
  vq_bus_2/1 -> d_vd_bus_2_block/2(State_vq_bus_2_07e0b), d_iq_line_8_2_block/2(State_vq_bus_2_12fee), vq_bus_2_out_block/1(State_vq_bus_2_798f2)
  d_vq_bus_9_block/1(Blockout_d_vq_bus_9_31261) -> vq_bus_9/1
  d_vq_bus_8_block/1(Blockout_d_vq_bus_8_09663) -> vq_bus_8/1
  d_id_line_7_8_block/1(Blockout_d_id_line_7_8_0c425) -> id_line_7_8/1
  d_id_load_5_block/1(Blockout_d_id_load_5_06c96) -> id_load_5/1
  d_id_load_9_block/1(Blockout_d_id_load_9_904a9) -> id_load_9/1
  d_iq_line_1_4_block/1(Blockout_d_iq_line_1_4_21ed7) -> iq_line_1_4/1
  d_iq_line_4_5_block/1(Blockout_d_iq_line_4_5_f0b45) -> iq_line_4_5/1
  d_iq_line_5_6_block/1(Blockout_d_iq_line_5_6_b9d91) -> iq_line_5_6/1
  d_iq_line_6_7_block/1(Blockout_d_iq_line_6_7_534ea) -> iq_line_6_7/1
  d_iq_load_7_block/1(Blockout_d_iq_load_7_bdd33) -> iq_load_7/1
  d_iq_line_8_9_block/1(Blockout_d_iq_line_8_9_5ccbd) -> iq_line_8_9/1
  d_iq_line_9_4_block/1(Blockout_d_iq_line_9_4_4ec5c) -> iq_line_9_4/1
  d_iq_load_9_block/1(Blockout_d_iq_load_9_4b775) -> iq_load_9/1
  d_vd_bus_8_block/1(Blockout_d_vd_bus_8_7183e) -> vd_bus_8/1
  d_vd_bus_1_block/1(Blockout_d_vd_bus_1_35ce7) -> vd_bus_1/1
  d_vd_bus_2_block/1(Blockout_d_vd_bus_2_06f1a) -> vd_bus_2/1
  d_vd_bus_3_block/1(Blockout_d_vd_bus_3_2695b) -> vd_bus_3/1
  d_vd_bus_5_block/1(Blockout_d_vd_bus_5_8bd9d) -> vd_bus_5/1
  d_vd_bus_6_block/1(Blockout_d_vd_bus_6_17a33) -> vd_bus_6/1
  d_vd_bus_7_block/1(Blockout_d_vd_bus_7_db642) -> vd_bus_7/1
  d_vd_bus_9_block/1(Blockout_d_vd_bus_9_ed3cf) -> vd_bus_9/1
  d_vq_bus_1_block/1(Blockout_d_vq_bus_1_47d83) -> vq_bus_1/1
  d_vq_bus_5_block/1(Blockout_d_vq_bus_5_ada7d) -> vq_bus_5/1
  d_vq_bus_6_block/1(Blockout_d_vq_bus_6_cdc68) -> vq_bus_6/1

== system case7/SG_D_1 ==
  v_d_SG_D_1 : Inport
  v_q_SG_D_1 : Inport  Port=2
  E_fd_SG_D_1 : Integrator  InitialCondition=1.886583745158506
  Px_1_SG_D_1 : Integrator  InitialCondition=0.0
  Px_2_SG_D_1 : Integrator  InitialCondition=0.0
  Px_3_SG_D_1 : Integrator  InitialCondition=-2.092721687039005e-24
  R_f_SG_D_1 : Integrator  InitialCondition=12.737135399455857
  T_e_SG_D_1_block : Subsystem
  T_m_SG_D_1 : Integrator  InitialCondition=0.7051405618875514
  V_f_SG_D_1 : Integrator  InitialCondition=18.865837451585058
  d_E_fd_SG_D_1_block : Subsystem
  d_Px_1_SG_D_1_block : Subsystem
  d_Px_2_SG_D_1_block : Subsystem
  d_Px_3_SG_D_1_block : Subsystem
  d_R_f_SG_D_1_block : Subsystem
  d_T_m_SG_D_1_block : Subsystem
  d_V_f_SG_D_1_block : Subsystem
  d_psi_1d_SG_D_1_block : Subsystem
  d_psi_d_SG_D_1_block : Subsystem
  d_psi_fd_SG_D_1_block : Subsystem
  d_psi_gq_SG_D_1_block : Subsystem
  d_psi_kq_SG_D_1_block : Subsystem
  d_psi_q_SG_D_1_block : Subsystem
  d_theta_SG_D_1_block : Subsystem
  d_w_SG_D_1_block : Subsystem
  i_d_SG_D_1_block : Subsystem
  i_q_SG_D_1_block : Subsystem
  psi_1d_SG_D_1 : Integrator  InitialCondition=0.8344526945464709
  psi_d_SG_D_1 : Integrator  InitialCondition=0.806016720205605
  psi_fd_SG_D_1 : Integrator  InitialCondition=0.9777700052244346
  psi_gq_SG_D_1 : Integrator  InitialCondition=0.365038146731613
  psi_kq_SG_D_1 : Integrator  InitialCondition=-0.5703721042681452
  psi_q_SG_D_1 : Integrator  InitialCondition=-0.5931869884388711
  theta_SG_D_1 : Integrator  InitialCondition=0.6342433928684046
  theta_SG_D_1_out_block : Subsystem
  w_SG_D_1 : Integrator  InitialCondition=376.99111843077515
  w_SG_D_1_out_block : Subsystem
  i_d_SG_D_1 : Outport
  i_q_SG_D_1 : Outport  Port=2
  T_e_SG_D_1 : Outport  Port=3
  w_SG_D_1_out : Outport  Port=4
  theta_SG_D_1_out : Outport  Port=5
  wires:
  T_m_SG_D_1/1 -> d_T_m_SG_D_1_block/2(State_T_m_SG_D_1_97fbd), d_w_SG_D_1_block/2(State_T_m_SG_D_1_54ed7)
  d_theta_SG_D_1_block/1(Blockout_d_theta_SG_D_1_2a112) -> theta_SG_D_1/1
  d_Px_1_SG_D_1_block/1(Blockout_d_Px_1_SG_D_1_d3439) -> Px_1_SG_D_1/1
  V_f_SG_D_1/1 -> d_V_f_SG_D_1_block/14(State_V_f_SG_D_1_6b3b6), d_E_fd_SG_D_1_block/2(State_V_f_SG_D_1_10c68)
  psi_kq_SG_D_1/1 -> d_psi_q_SG_D_1_block/2(State_psi_kq_SG_D_1_8ab4d), d_psi_gq_SG_D_1_block/3(State_psi_kq_SG_D_1_13776), d_psi_gq_SG_D_1_block/5(State_psi_kq_SG_D_1_16664), d_psi_kq_SG_D_1_block/4(State_psi_kq_SG_D_1_9c021), d_psi_kq_SG_D_1_block/2(State_psi_kq_SG_D_1_73ccc), d_w_SG_D_1_block/5(State_psi_kq_SG_D_1_738f2), i_d_SG_D_1_block/2(State_psi_kq_SG_D_1_5de85), i_q_SG_D_1_block/2(State_psi_kq_SG_D_1_2e921), d_V_f_SG_D_1_block/10(State_psi_kq_SG_D_1_f7694), d_psi_gq_SG_D_1_block/8(State_psi_kq_SG_D_1_82db5), T_e_SG_D_1_block/3(State_psi_kq_SG_D_1_0bf11)
  w_SG_D_1_out_block/1(Blockout_w_SG_D_1_out_64aa4) -> w_SG_D_1_out/1
  w_SG_D_1/1 -> d_psi_d_SG_D_1_block/9(State_w_SG_D_1_d723e), d_psi_q_SG_D_1_block/9(State_w_SG_D_1_b7eed), d_V_f_SG_D_1_block/13(State_w_SG_D_1_3f00e), d_w_SG_D_1_block/1(State_w_SG_D_1_87c27), d_Px_1_SG_D_1_block/2(State_w_SG_D_1_1213f), d_Px_2_SG_D_1_block/4(State_w_SG_D_1_9cb57), d_T_m_SG_D_1_block/1(State_w_SG_D_1_ed6bc), d_V_f_SG_D_1_block/8(State_w_SG_D_1_51b14), d_theta_SG_D_1_block/1(State_w_SG_D_1_8cf49), d_Px_3_SG_D_1_block/6(State_w_SG_D_1_58194), w_SG_D_1_out_block/1(State_w_SG_D_1_b6dd0)
  d_T_m_SG_D_1_block/1(Blockout_d_T_m_SG_D_1_03812) -> T_m_SG_D_1/1
  d_Px_3_SG_D_1_block/1(Blockout_d_Px_3_SG_D_1_d35bd) -> Px_3_SG_D_1/1
  d_Px_2_SG_D_1_block/1(Blockout_d_Px_2_SG_D_1_bbd82) -> Px_2_SG_D_1/1
  Px_2_SG_D_1/1 -> d_Px_3_SG_D_1_block/2(State_Px_2_SG_D_1_f74b9), d_Px_2_SG_D_1_block/1(State_Px_2_SG_D_1_00b8c), d_Px_3_SG_D_1_block/3(State_Px_2_SG_D_1_0b119)
  psi_q_SG_D_1/1 -> d_psi_q_SG_D_1_block/3(State_psi_q_SG_D_1_9b7b7), d_psi_gq_SG_D_1_block/6(State_psi_q_SG_D_1_f14e8), d_psi_gq_SG_D_1_block/9(State_psi_q_SG_D_1_8e0ca), d_psi_kq_SG_D_1_block/5(State_psi_q_SG_D_1_95dfc), d_w_SG_D_1_block/7(State_psi_q_SG_D_1_194a8), d_psi_d_SG_D_1_block/8(State_psi_q_SG_D_1_df331), d_w_SG_D_1_block/6(State_psi_q_SG_D_1_bda0b), d_V_f_SG_D_1_block/11(State_psi_q_SG_D_1_498a6), d_V_f_SG_D_1_block/7(State_psi_q_SG_D_1_1abe4), i_d_SG_D_1_block/3(State_psi_q_SG_D_1_bff72), i_q_SG_D_1_block/3(State_psi_q_SG_D_1_25865), T_e_SG_D_1_block/4(State_psi_q_SG_D_1_4e8fb), T_e_SG_D_1_block/5(State_psi_q_SG_D_1_74d13)
  v_q_SG_D_1/1 -> d_psi_q_SG_D_1_block/6(Input_v_q_SG_D_1_520ac), d_psi_d_SG_D_1_block/6(Input_v_q_SG_D_1_29a14)
  psi_fd_SG_D_1/1 -> d_psi_fd_SG_D_1_block/2(State_psi_fd_SG_D_1_89de8), d_psi_fd_SG_D_1_block/4(State_psi_fd_SG_D_1_3f013), d_psi_fd_SG_D_1_block/10(State_psi_fd_SG_D_1_d4d2a), d_psi_fd_SG_D_1_block/7(State_psi_fd_SG_D_1_23553), d_psi_d_SG_D_1_block/3(State_psi_fd_SG_D_1_b0bb2), d_psi_1d_SG_D_1_block/5(State_psi_fd_SG_D_1_e0875), d_w_SG_D_1_block/10(State_psi_fd_SG_D_1_43345), i_d_SG_D_1_block/7(State_psi_fd_SG_D_1_7462f), d_psi_1d_SG_D_1_block/2(State_psi_fd_SG_D_1_1ada6), d_V_f_SG_D_1_block/6(State_psi_fd_SG_D_1_514a1), i_q_SG_D_1_block/7(State_psi_fd_SG_D_1_21903), T_e_SG_D_1_block/8(State_psi_fd_SG_D_1_5c3bd)
  psi_gq_SG_D_1/1 -> d_psi_q_SG_D_1_block/1(State_psi_gq_SG_D_1_4f3e1), d_psi_gq_SG_D_1_block/1(State_psi_gq_SG_D_1_444f1), d_psi_gq_SG_D_1_block/2(State_psi_gq_SG_D_1_57806), d_psi_gq_SG_D_1_block/4(State_psi_gq_SG_D_1_08786), d_psi_gq_SG_D_1_block/7(State_psi_gq_SG_D_1_7ad27), d_psi_kq_SG_D_1_block/3(State_psi_gq_SG_D_1_32f50), d_psi_kq_SG_D_1_block/1(State_psi_gq_SG_D_1_141c0), d_w_SG_D_1_block/4(State_psi_gq_SG_D_1_c9957), d_V_f_SG_D_1_block/9(State_psi_gq_SG_D_1_81dd7), i_d_SG_D_1_block/1(State_psi_gq_SG_D_1_613ce), i_q_SG_D_1_block/1(State_psi_gq_SG_D_1_d72fd), T_e_SG_D_1_block/2(State_psi_gq_SG_D_1_d5669)
  v_d_SG_D_1/1 -> d_psi_d_SG_D_1_block/4(Input_v_d_SG_D_1_36932), d_psi_q_SG_D_1_block/4(Input_v_d_SG_D_1_5bf66)
  theta_SG_D_1/1 -> d_psi_d_SG_D_1_block/5(State_theta_SG_D_1_2d59f), d_psi_q_SG_D_1_block/5(State_theta_SG_D_1_45d91), d_psi_d_SG_D_1_block/7(State_theta_SG_D_1_b3d69), d_psi_q_SG_D_1_block/7(State_theta_SG_D_1_c7f9c), i_d_SG_D_1_block/4(State_theta_SG_D_1_6929e), i_d_SG_D_1_block/8(State_theta_SG_D_1_df07b), i_q_SG_D_1_block/4(State_theta_SG_D_1_37866), i_q_SG_D_1_block/8(State_theta_SG_D_1_2b1c8), theta_SG_D_1_out_block/1(State_theta_SG_D_1_a05eb)
  psi_d_SG_D_1/1 -> d_psi_fd_SG_D_1_block/6(State_psi_d_SG_D_1_6490f), d_psi_q_SG_D_1_block/8(State_psi_d_SG_D_1_d17e6), d_psi_1d_SG_D_1_block/4(State_psi_d_SG_D_1_1ea7c), d_psi_fd_SG_D_1_block/9(State_psi_d_SG_D_1_0357b), d_V_f_SG_D_1_block/5(State_psi_d_SG_D_1_2b785), d_V_f_SG_D_1_block/12(State_psi_d_SG_D_1_17f8b), i_d_SG_D_1_block/6(State_psi_d_SG_D_1_04ecd), i_q_SG_D_1_block/6(State_psi_d_SG_D_1_25480), d_w_SG_D_1_block/9(State_psi_d_SG_D_1_5b665), d_w_SG_D_1_block/3(State_psi_d_SG_D_1_2b637), T_e_SG_D_1_block/1(State_psi_d_SG_D_1_a3ce0), d_psi_d_SG_D_1_block/2(State_psi_d_SG_D_1_516f9), T_e_SG_D_1_block/7(State_psi_d_SG_D_1_70569)
  d_E_fd_SG_D_1_block/1(Blockout_d_E_fd_SG_D_1_39807) -> E_fd_SG_D_1/1
  psi_1d_SG_D_1/1 -> d_psi_fd_SG_D_1_block/3(State_psi_1d_SG_D_1_80808), d_psi_fd_SG_D_1_block/5(State_psi_1d_SG_D_1_e7af2), d_psi_fd_SG_D_1_block/8(State_psi_1d_SG_D_1_8dc8e), d_psi_d_SG_D_1_block/1(State_psi_1d_SG_D_1_721c9), d_psi_1d_SG_D_1_block/1(State_psi_1d_SG_D_1_e7f45), d_psi_1d_SG_D_1_block/3(State_psi_1d_SG_D_1_ed62b), d_V_f_SG_D_1_block/4(State_psi_1d_SG_D_1_2c4ca), i_d_SG_D_1_block/5(State_psi_1d_SG_D_1_bfd03), i_q_SG_D_1_block/5(State_psi_1d_SG_D_1_f3b13), d_w_SG_D_1_block/8(State_psi_1d_SG_D_1_0f07b), T_e_SG_D_1_block/6(State_psi_1d_SG_D_1_b5c2d)
  Px_1_SG_D_1/1 -> d_Px_1_SG_D_1_block/1(State_Px_1_SG_D_1_12f8b), d_Px_2_SG_D_1_block/2(State_Px_1_SG_D_1_dc188), d_Px_3_SG_D_1_block/4(State_Px_1_SG_D_1_9c31b), d_Px_3_SG_D_1_block/5(State_Px_1_SG_D_1_3806b), d_Px_2_SG_D_1_block/3(State_Px_1_SG_D_1_61a1c)
  d_psi_gq_SG_D_1_block/1(Blockout_d_psi_gq_SG_D_1_67353) -> psi_gq_SG_D_1/1
  d_psi_q_SG_D_1_block/1(Blockout_d_psi_q_SG_D_1_cd2a8) -> psi_q_SG_D_1/1
  d_w_SG_D_1_block/1(Blockout_d_w_SG_D_1_ca62c) -> w_SG_D_1/1
  d_psi_kq_SG_D_1_block/1(Blockout_d_psi_kq_SG_D_1_55298) -> psi_kq_SG_D_1/1
  d_V_f_SG_D_1_block/1(Blockout_d_V_f_SG_D_1_27703) -> V_f_SG_D_1/1
  T_e_SG_D_1_block/1(Blockout_T_e_SG_D_1_7d4c7) -> T_e_SG_D_1/1
  i_q_SG_D_1_block/1(Blockout_i_q_SG_D_1_6d7e3) -> i_q_SG_D_1/1
  i_d_SG_D_1_block/1(Blockout_i_d_SG_D_1_6a835) -> i_d_SG_D_1/1
  d_R_f_SG_D_1_block/1(Blockout_d_R_f_SG_D_1_0120a) -> R_f_SG_D_1/1
  theta_SG_D_1_out_block/1(Blockout_theta_SG_D_1_out_771f4) -> theta_SG_D_1_out/1
  d_psi_d_SG_D_1_block/1(Blockout_d_psi_d_SG_D_1_499f8) -> psi_d_SG_D_1/1
  d_psi_1d_SG_D_1_block/1(Blockout_d_psi_1d_SG_D_1_e2098) -> psi_1d_SG_D_1/1
  R_f_SG_D_1/1 -> d_V_f_SG_D_1_block/2(State_R_f_SG_D_1_bc712), d_R_f_SG_D_1_block/2(State_R_f_SG_D_1_306fb)
  Px_3_SG_D_1/1 -> d_V_f_SG_D_1_block/3(State_Px_3_SG_D_1_d93e1), d_Px_3_SG_D_1_block/1(State_Px_3_SG_D_1_1460f)
  E_fd_SG_D_1/1 -> d_V_f_SG_D_1_block/1(State_E_fd_SG_D_1_3a6c9), d_R_f_SG_D_1_block/1(State_E_fd_SG_D_1_6cf46), d_E_fd_SG_D_1_block/1(State_E_fd_SG_D_1_10d5b), d_psi_fd_SG_D_1_block/1(State_E_fd_SG_D_1_9c11e)
  d_psi_fd_SG_D_1_block/1(Blockout_d_psi_fd_SG_D_1_20036) -> psi_fd_SG_D_1/1
